simulink model "V2V"  (R2023a)
settings: Solver=FixedStepDiscrete  StartTime=0.0  StopTime=10  FixedStep=0.1  RelTol=1e-3
undefined symbols (not defined in the file): samp_time
(part 1 of 2)
settings Model: Creator=maurizio  LastModifiedBy=alessio
settings SolverCC: MinimalZcImpactIntegration=on
settings DebuggingCC: ReadBeforeWriteMsg=DisableAll  WriteAfterWriteMsg=DisableAll  WriteAfterReadMsg=DisableAll  MultiTaskDSMMsg=none  ModelReferenceSymbolNameMessage=none
settings HardwareCC: TargetBitPerLong=64  TargetBitPerPointer=64  TargetBitPerSizeT=64  TargetBitPerPtrDiffT=64  TargetLongLongMode=on  TargetIntDivRoundTo=Zero  TargetEndianess=LittleEndian  TargetWordSize=64  TargetHWDeviceType=MATLAB Host  ProdEqTarget=off
settings ModelReferenceCC: UpdateModelReferenceTargets=IfOutOfDate
settings SFSimCC: SFSimEcho=off
settings RTWCC: Description=FMU2CS  SystemTargetFile=fmu2cs.tlc  TemplateMakefile=fmu2cs_default_tmf  RTWVerbose=off  RTWUseSimCustomCode=on  BuildConfiguration=Faster Runs
settings CodeAppCC: MaxIdLength=255
settings FMU2CSTargetCC: TargetFcnLib=ansi_tfl_table_tmw.mat  GenFloatMathFcnCalls=NOT IN USE  TargetLangStandard=C99 (ISO)  CodeReplacementLibrary=None  UtilityFuncGeneration=Auto  MultiwordTypeDef=System defined  MultiwordLength=2048  DynamicStringBufferSize=256  GenerateFullHeader=on  InferredTypesCompatibility=off  GenerateSampleERTMain=off  GenerateTestInterfaces=off  ModelReferenceCompliant=on  ParMdlRefBuildCompliant=on  CompOptLevelCompliant=on  ConcurrentExecutionCompliant=on  IncludeMdlTerminateFcn=on  CombineOutputUpdateFcns=on  CombineSignalStateStructs=off  GroupInternalDataByFunction=off  SuppressErrorStatus=off  IncludeFileDelimiter=Auto  ERTCustomFileBanners=off  SupportAbsoluteTime=on  LogVarNameModifier=rt_  MatFileLogging=off  CodeInterfacePackaging=Nonreusable function  PurelyIntegerCode=off  SupportNonFinite=on  SupportComplex=on  SupportContinuousTime=on  SupportNonInlinedSFcns=on  RemoveDisableFunc=off  RemoveResetFunc=off  SupportVariableSizeSignals=off  ParenthesesLevel=Nominal  CastingMode=Nominal  MATLABClassNameForMDSCustomization=Simulink.SoftwareTarget.GRTCustomization  ModelStepFunctionPrototypeControlCompliant=off  CPPClassGenCompliant=on  AutosarCompliant=off  MDXCompliant=off  GRTInterface=off  GenerateAllocFcn=off  UseToolchainInfoCompliant=on  GenerateSharedConstants=on  CoderGroups=[]  AccessMethods=[]  LookupTableObjectStructAxisOrder=1,2,3,4,...  LUTObjectStructOrderExplicitValues=Size,Breakpoints,Table  LUTObjectStructOrderEvenSpacing=Size,Breakpoints,Table  ArrayLayout=Column-major  UnsupportedSFcnMsg=error  ERTHeaderFileRootName=$R$E  ERTSourceFileRootName=$R$E  ERTDataFileRootName=$R_data  OptimizeReductions=off  UseMalloc=off  ExtMode=off  ExtModeStaticAlloc=off  ExtModeTesting=off  ExtModeAutomaticAllocSize=on  ExtModeMaxTrigDuration=10  ExtModeStaticAllocSize=1000000  ExtModeTransport=0  ExtModeMexFile=ext_comm  ExtModeIntrfLevel=Level1  RTWCAPISignals=off  RTWCAPIParams=off  RTWCAPIStates=off  RTWCAPIRootIO=off  GenerateASAP2=off  MultiInstanceErrorCode=Error  CreateModelAfterGeneratingFMU=on  ExportedContent=project  ProjectName=off  AddIcon=off  SaveSourceCodeToFMU=off  AddNativeSimulinkBehavior=off  DataTypeConversion=off  GenerateLinuxBinaryWithWSL=off  FMUType=CS  FMIVersion=2

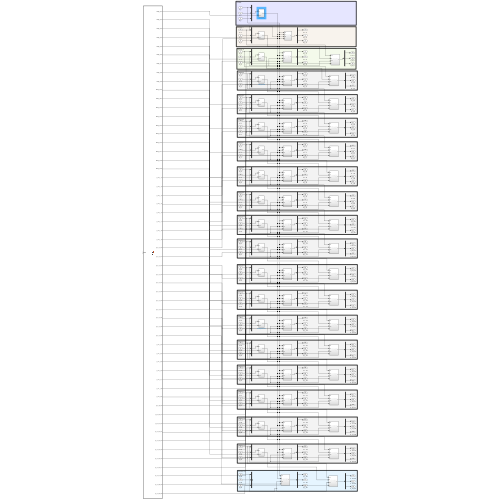
[thumbnail: Simulink's stored preview of the top-level diagram]
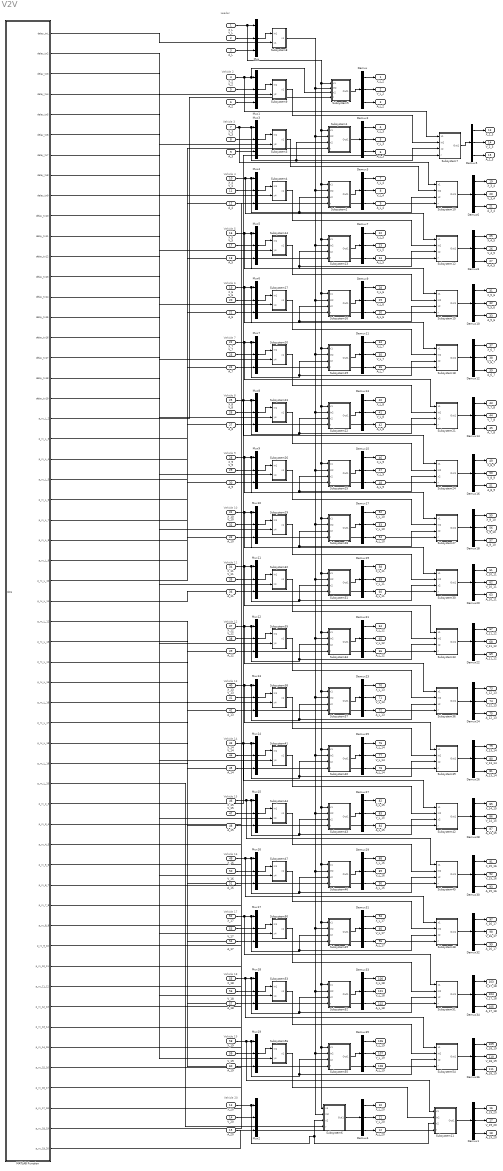
== system V2V ==
  note: Vehicle 3
  note: Vehicle 20
  note: Vehicle 4
  note: Vehicle 2
  note: Leader
  note: Vehicle 5
  note: Vehicle 6
  note: Vehicle 7
  note: Vehicle 8
  note: Vehicle 9
  note: Vehicle 10
  note: Vehicle 11
  note: Vehicle 12
  note: Vehicle 13
  note: Vehicle 14
  note: Vehicle 15
  note: Vehicle 16
  note: Vehicle 17
  note: Vehicle 18
  note: Vehicle 19
  X_L : Inport
  V_L : Inport  Port=2
  A_L : Inport  Port=3
  X_2 : Inport  Port=4
  V_2 : Inport  Port=5
  A_2 : Inport  Port=6
  X_3 : Inport  Port=7
  V_3 : Inport  Port=8
  A_3 : Inport  Port=9
  X_4 : Inport  Port=10
  V_4 : Inport  Port=11
  A_4 : Inport  Port=12
  X_20 : Inport  Port=13
  V_20 : Inport  Port=14
  A_20 : Inport  Port=15
  X_5 : Inport  Port=16
  V_5 : Inport  Port=17
  A_5 : Inport  Port=18
  X_6 : Inport  Port=19
  V_6 : Inport  Port=20
  A_6 : Inport  Port=21
  X_7 : Inport  Port=22
  V_7 : Inport  Port=23
  A_7 : Inport  Port=24
  X_8 : Inport  Port=25
  V_8 : Inport  Port=26
  A_8 : Inport  Port=27
  X_9 : Inport  Port=28
  V_9 : Inport  Port=29
  A_9 : Inport  Port=30
  X_10 : Inport  Port=31
  V_10 : Inport  Port=32
  A_10 : Inport  Port=33
  X_11 : Inport  Port=34
  V_11 : Inport  Port=35
  A_11 : Inport  Port=36
  X_12 : Inport  Port=37
  V_12 : Inport  Port=38
  A_12 : Inport  Port=39
  X_13 : Inport  Port=40
  V_13 : Inport  Port=41
  A_13 : Inport  Port=42
  X_14 : Inport  Port=43
  V_14 : Inport  Port=44
  A_14 : Inport  Port=45
  X_15 : Inport  Port=46
  V_15 : Inport  Port=47
  A_15 : Inport  Port=48
  X_16 : Inport  Port=49
  V_16 : Inport  Port=50
  A_16 : Inport  Port=51
  X_17 : Inport  Port=52
  V_17 : Inport  Port=53
  A_17 : Inport  Port=54
  X_18 : Inport  Port=55
  V_18 : Inport  Port=56
  A_18 : Inport  Port=57
  X_19 : Inport  Port=58
  V_19 : Inport  Port=59
  A_19 : Inport  Port=60
  Demux{,1..36} (37 alike) : Demux  Outputs=3
  MATLAB Function : MATLAB Function  TreatAsAtomicUnit=on  SystemSampleTime=0.1
  Mux{,1..19} (20 alike) : Mux  Inputs=3
  Subsystem1 : Subsystem
  Subsystem10 : Subsystem
  Subsystem11 : Subsystem
  Subsystem12 : Subsystem
  Subsystem13 : Subsystem
  Subsystem14 : Subsystem
  Subsystem15 : Subsystem
  Subsystem16 : Subsystem
  Subsystem17 : Subsystem
  Subsystem18 : Subsystem
  Subsystem19 : Subsystem
  Subsystem2 : Subsystem
  Subsystem20 : Subsystem
  Subsystem21 : Subsystem
  Subsystem22 : Subsystem
  Subsystem23 : Subsystem
  Subsystem24 : Subsystem
  Subsystem25 : Subsystem
  Subsystem26 : Subsystem
  Subsystem27 : Subsystem
  Subsystem28 : Subsystem
  Subsystem29 : Subsystem
  Subsystem3 : Subsystem
  Subsystem30 : Subsystem
  Subsystem31 : Subsystem
  Subsystem32 : Subsystem
  Subsystem33 : Subsystem
  Subsystem34 : Subsystem
  Subsystem35 : Subsystem
  Subsystem36 : Subsystem
  Subsystem37 : Subsystem
  Subsystem38 : Subsystem
  Subsystem39 : Subsystem
  Subsystem4 : Subsystem
  Subsystem40 : Subsystem
  Subsystem41 : Subsystem
  Subsystem42 : Subsystem
  Subsystem43 : Subsystem
  Subsystem44 : Subsystem
  Subsystem45 : Subsystem
  Subsystem46 : Subsystem
  Subsystem47 : Subsystem
  Subsystem48 : Subsystem
  Subsystem49 : Subsystem
  Subsystem5 : Subsystem
  Subsystem50 : Subsystem
  Subsystem51 : Subsystem
  Subsystem52 : Subsystem
  Subsystem53 : Subsystem
  Subsystem54 : Subsystem
  Subsystem55 : Subsystem
  Subsystem56 : Subsystem
  Subsystem6 : Subsystem
  Subsystem7 : Subsystem
  Subsystem8 : Subsystem
  Subsystem9 : Subsystem
  X_L_2 : Outport
  V_L_2 : Outport  Port=2
  A_L_2 : Outport  Port=3
  X_L_3 : Outport  Port=4
  V_L_3 : Outport  Port=5
  A_L_3 : Outport  Port=6
  X_L_4 : Outport  Port=7
  V_L_4 : Outport  Port=8
  A_L_4 : Outport  Port=9
  X_L_20 : Outport  Port=10
  V_L_20 : Outport  Port=11
  A_L_20 : Outport  Port=12
  X_2_3 : Outport  Port=13
  V_2_3 : Outport  Port=14
  A_2_3 : Outport  Port=15
  X_19_20 : Outport  Port=16
  V_19_20 : Outport  Port=17
  A_19_20 : Outport  Port=18
  X_3_4 : Outport  Port=19
  V_3_4 : Outport  Port=20
  A_3_4 : Outport  Port=21
  X_L_5 : Outport  Port=22
  V_L_5 : Outport  Port=23
  A_L_5 : Outport  Port=24
  X_4_5 : Outport  Port=25
  V_4_5 : Outport  Port=26
  A_4_5 : Outport  Port=27
  X_L_6 : Outport  Port=28
  V_L_6 : Outport  Port=29
  A_L_6 : Outport  Port=30
  X_5_6 : Outport  Port=31
  V_5_6 : Outport  Port=32
  A_5_6 : Outport  Port=33
  X_L_7 : Outport  Port=34
  V_L_7 : Outport  Port=35
  A_L_7 : Outport  Port=36
  X_6_7 : Outport  Port=37
  V_6_7 : Outport  Port=38
  A_6_7 : Outport  Port=39
  X_L_8 : Outport  Port=40
  V_L_8 : Outport  Port=41
  A_L_8 : Outport  Port=42
  X_7_8 : Outport  Port=43
  V_7_8 : Outport  Port=44
  A_7_8 : Outport  Port=45
  X_L_9 : Outport  Port=46
  V_L_9 : Outport  Port=47
  A_L_9 : Outport  Port=48
  X_8_9 : Outport  Port=49
  V_8_9 : Outport  Port=50
  A_8_9 : Outport  Port=51
  X_L_10 : Outport  Port=52
  V_L_10 : Outport  Port=53
  A_L_10 : Outport  Port=54
  X_9_10 : Outport  Port=55
  V_9_10 : Outport  Port=56
  A_9_10 : Outport  Port=57
  X_L_11 : Outport  Port=58
  V_L_11 : Outport  Port=59
  A_L_11 : Outport  Port=60
  X_10_11 : Outport  Port=61
  V_10_11 : Outport  Port=62
  A_10_11 : Outport  Port=63
  X_L_12 : Outport  Port=64
  V_L_12 : Outport  Port=65
  A_L_12 : Outport  Port=66
  X_11_12 : Outport  Port=67
  V_11_12 : Outport  Port=68
  A_11_12 : Outport  Port=69
  X_L_13 : Outport  Port=70
  V_L_13 : Outport  Port=71
  A_L_13 : Outport  Port=72
  X_12_13 : Outport  Port=73
  V_12_13 : Outport  Port=74
  A_12_13 : Outport  Port=75
  X_L_14 : Outport  Port=76
  V_L_14 : Outport  Port=77
  A_L_14 : Outport  Port=78
  X_13_14 : Outport  Port=79
  V_13_14 : Outport  Port=80
  A_13_14 : Outport  Port=81
  X_L_15 : Outport  Port=82
  V_L_15 : Outport  Port=83
  A_L_15 : Outport  Port=84
  X_14_15 : Outport  Port=85
  V_14_15 : Outport  Port=86
  A_14_15 : Outport  Port=87
  X_L_16 : Outport  Port=88
  V_L_16 : Outport  Port=89
  A_L_16 : Outport  Port=90
  X_15_16 : Outport  Port=91
  V_15_16 : Outport  Port=92
  A_15_16 : Outport  Port=93
  X_L_17 : Outport  Port=94
  V_L_17 : Outport  Port=95
  A_L_17 : Outport  Port=96
  X_16_17 : Outport  Port=97
  V_16_17 : Outport  Port=98
  A_16_17 : Outport  Port=99
  X_L_18 : Outport  Port=100
  V_L_18 : Outport  Port=101
  A_L_18 : Outport  Port=102
  X_17_18 : Outport  Port=103
  V_17_18 : Outport  Port=104
  A_17_18 : Outport  Port=105
  X_L_19 : Outport  Port=106
  V_L_19 : Outport  Port=107
  A_L_19 : Outport  Port=108
  X_18_19 : Outport  Port=109
  V_18_19 : Outport  Port=110
  A_18_19 : Outport  Port=111
  wires:
  V_L/1 -> Mux/2
  X_L/1 -> Subsystem5/1(x1), Subsystem6/1(x1), Subsystem55/1(x1), Subsystem52/1(x1), Subsystem49/1(x1), Subsystem46/1(x1), Subsystem43/1(x1), Subsystem40/1(x1), Subsystem37/1(x1), Subsystem34/1(x1), Subsystem31/1(x1), Subsystem28/1(x1), Subsystem25/1(x1), Subsystem22/1(x1), Subsystem19/1(x1), Subsystem16/1(x1), Subsystem13/1(x1), Subsystem2/1(x1), Subsystem1/1(x1), Mux/1
  A_L/1 -> Mux/3
  X_2/1 -> Subsystem7/1(x1), Subsystem5/3(x2), Mux1/1
  V_2/1 -> Mux1/2
  A_2/1 -> Mux1/3
  A_3/1 -> Mux3/3
  V_3/1 -> Mux3/2
  X_4/1 -> Subsystem12/1(x1), Subsystem10/3(x2), Subsystem2/3(x2), Mux4/1
  A_4/1 -> Mux4/3
  X_3/1 -> Subsystem10/1(x1), Subsystem7/3(x2), Subsystem1/3(x2), Mux3/1
  V_4/1 -> Mux4/2
  Demux/1 -> X_L_2/1
  Demux/2 -> V_L_2/1
  Demux/3 -> A_L_2/1
  Demux2/1 -> X_L_3/1
  Demux2/3 -> A_L_3/1
  Demux2/2 -> V_L_3/1
  Demux3/3 -> A_L_4/1
  Demux3/1 -> X_L_4/1
  Demux3/2 -> V_L_4/1
  Demux4/2 -> V_L_20/1
  Demux4/1 -> X_L_20/1
  Demux4/3 -> A_L_20/1
  Demux5/3 -> A_2_3/1
  Demux5/2 -> V_2_3/1
  Demux5/1 -> X_2_3/1
  Demux1/3 -> A_19_20/1
  Demux1/2 -> V_19_20/1
  Demux1/1 -> X_19_20/1
  Demux6/3 -> A_3_4/1
  Demux6/2 -> V_3_4/1
  Demux6/1 -> X_3_4/1
  Mux1/1 -> Subsystem9/1(In1)
  Mux3/1 -> Subsystem3/1(In1)
  Mux4/1 -> Subsystem4/1(In1)
  Subsystem5/1(Out1) -> Demux/1
  Mux/1 -> Subsystem8/1(In1)
  Subsystem8/1(x1) -> Subsystem6/2(In2), Subsystem55/2(In2), Subsystem52/2(In2), Subsystem49/2(In2), Subsystem46/2(In2), Subsystem43/2(In2), Subsystem40/2(In2), Subsystem37/2(In2), Subsystem34/2(In2), Subsystem31/2(In2), Subsystem28/2(In2), Subsystem25/2(In2), Subsystem22/2(In2), Subsystem19/2(In2), Subsystem16/2(In2), Subsystem13/2(In2), Subsystem2/2(In2), Subsystem1/2(In2), Subsystem5/2(In2)
  Subsystem2/1(Out1) -> Demux3/1
  Subsystem6/1(Out1) -> Demux4/1
  V_20/1 -> Mux2/2
  A_20/1 -> Mux2/3
  X_20/1 -> Subsystem11/3(x2), Subsystem6/3(x2), Mux2/1
  Subsystem1/1(Out1) -> Demux2/1
  Subsystem7/1(Out1) -> Demux5/1
  Subsystem10/1(Out1) -> Demux6/1
  Subsystem11/1(Out1) -> Demux1/1
  Subsystem9/1(x1) -> Subsystem7/2(In2)
  Subsystem3/1(x1) -> Subsystem10/2(In2)
  MATLAB Function/1(delay_txL) -> Subsystem8/2(y1)
  MATLAB Function/2(delay_tx2) -> Subsystem9/2(y2)
  MATLAB Function/3(delay_tx3) -> Subsystem3/2(y3)
  MATLAB Function/4(delay_tx4) -> Subsystem4/2(y4)
  A_5/1 -> Mux5/3
  Demux7/1 -> X_L_5/1
  Demux7/2 -> V_L_5/1
  Demux7/3 -> A_L_5/1
  Subsystem12/1(Out1) -> Demux8/1
  X_5/1 -> Subsystem15/1(x1), Subsystem12/3(x2), Subsystem13/3(x2), Mux5/1
  Demux8/3 -> A_4_5/1
  V_5/1 -> Mux5/2
  Subsystem13/1(Out1) -> Demux7/1
  Demux8/1 -> X_4_5/1
  Mux5/1 -> Subsystem14/1(In1)
  Demux8/2 -> V_4_5/1
  Subsystem16/1(Out1) -> Demux9/1
  Demux9/3 -> A_L_6/1
  V_6/1 -> Mux6/2
  Demux10/3 -> A_5_6/1
  Demux10/2 -> V_5_6/1
  A_6/1 -> Mux6/3
  X_6/1 -> Subsystem18/1(x1), Subsystem15/3(x2), Subsystem16/3(x2), Mux6/1
  Mux6/1 -> Subsystem17/1(In1)
  Subsystem15/1(Out1) -> Demux10/1
  Demux9/1 -> X_L_6/1
  Demux9/2 -> V_L_6/1
  Demux10/1 -> X_5_6/1
  Subsystem19/1(Out1) -> Demux11/1
  Demux11/3 -> A_L_7/1
  V_7/1 -> Mux7/2
  Demux12/3 -> A_6_7/1
  Demux12/2 -> V_6_7/1
  A_7/1 -> Mux7/3
  X_7/1 -> Subsystem21/1(x1), Subsystem18/3(x2), Subsystem19/3(x2), Mux7/1
  Mux7/1 -> Subsystem20/1(In1)
  Subsystem18/1(Out1) -> Demux12/1
  Demux11/1 -> X_L_7/1
  Demux11/2 -> V_L_7/1
  Demux12/1 -> X_6_7/1
  Subsystem22/1(Out1) -> Demux13/1
  Demux13/3 -> A_L_8/1
  V_8/1 -> Mux8/2
  Demux14/3 -> A_7_8/1
  Demux14/2 -> V_7_8/1
  A_8/1 -> Mux8/3
  X_8/1 -> Subsystem24/1(x1), Subsystem21/3(x2), Subsystem22/3(x2), Mux8/1
  Mux8/1 -> Subsystem23/1(In1)
  Subsystem21/1(Out1) -> Demux14/1
  Demux13/1 -> X_L_8/1
  Demux13/2 -> V_L_8/1
  Demux14/1 -> X_7_8/1
  Subsystem25/1(Out1) -> Demux15/1
  Demux15/3 -> A_L_9/1
  V_9/1 -> Mux9/2
  Demux16/3 -> A_8_9/1
  Demux16/2 -> V_8_9/1
  A_9/1 -> Mux9/3
  X_9/1 -> Subsystem27/1(x1), Subsystem24/3(x2), Subsystem25/3(x2), Mux9/1
  Mux9/1 -> Subsystem26/1(In1)
  Subsystem24/1(Out1) -> Demux16/1
  Demux15/1 -> X_L_9/1
  Demux15/2 -> V_L_9/1
  Demux16/1 -> X_8_9/1
  Subsystem28/1(Out1) -> Demux17/1
  Demux17/3 -> A_L_10/1
  V_10/1 -> Mux10/2
  Demux18/3 -> A_9_10/1
  Demux18/2 -> V_9_10/1
  A_10/1 -> Mux10/3
  X_10/1 -> Subsystem30/1(x1), Subsystem27/3(x2), Subsystem28/3(x2), Mux10/1
  Mux10/1 -> Subsystem29/1(In1)
  Subsystem27/1(Out1) -> Demux18/1
  Demux17/1 -> X_L_10/1
  Demux17/2 -> V_L_10/1
  Demux18/1 -> X_9_10/1
  Subsystem31/1(Out1) -> Demux19/1
  Demux19/3 -> A_L_11/1
  V_11/1 -> Mux11/2
  Demux20/3 -> A_10_11/1
  Demux20/2 -> V_10_11/1
  A_11/1 -> Mux11/3
  X_11/1 -> Subsystem33/1(x1), Subsystem30/3(x2), Subsystem31/3(x2), Mux11/1
  Mux11/1 -> Subsystem32/1(In1)
  Subsystem30/1(Out1) -> Demux20/1
  Demux19/1 -> X_L_11/1
  Demux19/2 -> V_L_11/1
  Demux20/1 -> X_10_11/1
  Subsystem34/1(Out1) -> Demux21/1
  Demux21/3 -> A_L_12/1
  V_12/1 -> Mux12/2
  Demux22/3 -> A_11_12/1
  Demux22/2 -> V_11_12/1
  A_12/1 -> Mux12/3
  X_12/1 -> Subsystem36/1(x1), Subsystem33/3(x2), Subsystem34/3(x2), Mux12/1
  Mux12/1 -> Subsystem35/1(In1)
  Subsystem33/1(Out1) -> Demux22/1
  Demux21/1 -> X_L_12/1
  Demux21/2 -> V_L_12/1
  Demux22/1 -> X_11_12/1
  Subsystem37/1(Out1) -> Demux23/1
  Demux23/3 -> A_L_13/1
  V_13/1 -> Mux13/2
  Demux24/3 -> A_12_13/1
  Demux24/2 -> V_12_13/1
  A_13/1 -> Mux13/3
  X_13/1 -> Subsystem39/1(x1), Subsystem36/3(x2), Subsystem37/3(x2), Mux13/1
  Mux13/1 -> Subsystem38/1(In1)
  Subsystem36/1(Out1) -> Demux24/1
  Demux23/1 -> X_L_13/1
  Demux23/2 -> V_L_13/1
  Demux24/1 -> X_12_13/1
  Subsystem40/1(Out1) -> Demux25/1
  Demux25/3 -> A_L_14/1
  V_14/1 -> Mux14/2
  Demux26/3 -> A_13_14/1
  Demux26/2 -> V_13_14/1
  A_14/1 -> Mux14/3
  X_14/1 -> Subsystem42/1(x1), Subsystem39/3(x2), Subsystem40/3(x2), Mux14/1
  Mux14/1 -> Subsystem41/1(In1)
  Subsystem39/1(Out1) -> Demux26/1
  Demux25/1 -> X_L_14/1
  Demux25/2 -> V_L_14/1
  Demux26/1 -> X_13_14/1
  Subsystem43/1(Out1) -> Demux27/1
  Demux27/3 -> A_L_15/1
  V_15/1 -> Mux15/2
  Demux28/3 -> A_14_15/1
  Demux28/2 -> V_14_15/1
  A_15/1 -> Mux15/3
  X_15/1 -> Subsystem45/1(x1), Subsystem42/3(x2), Subsystem43/3(x2), Mux15/1
  Mux15/1 -> Subsystem44/1(In1)
  Subsystem42/1(Out1) -> Demux28/1
  Demux27/1 -> X_L_15/1
  Demux27/2 -> V_L_15/1
  Demux28/1 -> X_14_15/1
  Subsystem46/1(Out1) -> Demux29/1
  Demux29/3 -> A_L_16/1
  V_16/1 -> Mux16/2
  Demux30/3 -> A_15_16/1
  Demux30/2 -> V_15_16/1
  A_16/1 -> Mux16/3
  X_16/1 -> Subsystem48/1(x1), Subsystem45/3(x2), Subsystem46/3(x2), Mux16/1
  Mux16/1 -> Subsystem47/1(In1)
  Subsystem45/1(Out1) -> Demux30/1
  Demux29/1 -> X_L_16/1
  Demux29/2 -> V_L_16/1
  Demux30/1 -> X_15_16/1
  Subsystem49/1(Out1) -> Demux31/1
  Demux31/3 -> A_L_17/1
  V_17/1 -> Mux17/2
  Demux32/3 -> A_16_17/1
  Demux32/2 -> V_16_17/1
  A_17/1 -> Mux17/3
  X_17/1 -> Subsystem51/1(x1), Subsystem48/3(x2), Subsystem49/3(x2), Mux17/1
  Mux17/1 -> Subsystem50/1(In1)
  Subsystem48/1(Out1) -> Demux32/1
  Demux31/1 -> X_L_17/1
  Demux31/2 -> V_L_17/1
  Demux32/1 -> X_16_17/1
  Subsystem52/1(Out1) -> Demux33/1
  Demux33/3 -> A_L_18/1
  V_18/1 -> Mux18/2
  Demux34/3 -> A_17_18/1
  Demux34/2 -> V_17_18/1
  A_18/1 -> Mux18/3
  X_18/1 -> Subsystem54/1(x1), Subsystem51/3(x2), Subsystem52/3(x2), Mux18/1
  Mux18/1 -> Subsystem53/1(In1)
  Subsystem51/1(Out1) -> Demux34/1
  Demux33/1 -> X_L_18/1
  Demux33/2 -> V_L_18/1
  Demux34/1 -> X_17_18/1
  Subsystem55/1(Out1) -> Demux35/1
  Demux35/3 -> A_L_19/1
  V_19/1 -> Mux19/2
  Demux36/3 -> A_18_19/1
  Demux36/2 -> V_18_19/1
  A_19/1 -> Mux19/3
  X_19/1 -> Subsystem11/1(x1), Subsystem54/3(x2), Subsystem55/3(x2), Mux19/1
  Mux19/1 -> Subsystem56/1(In1)
  Subsystem54/1(Out1) -> Demux36/1
  Demux35/1 -> X_L_19/1
  Demux35/2 -> V_L_19/1
  Demux36/1 -> X_18_19/1
  MATLAB Function/5(delay_tx5) -> Subsystem14/2(y4)
  MATLAB Function/6(delay_tx6) -> Subsystem17/2(y4)
  MATLAB Function/7(delay_tx7) -> Subsystem20/2(y4)
  MATLAB Function/8(delay_tx8) -> Subsystem23/2(y4)
  MATLAB Function/9(delay_tx9) -> Subsystem26/2(y4)
  MATLAB Function/10(delay_tx10) -> Subsystem29/2(y4)
  MATLAB Function/11(delay_tx11) -> Subsystem32/2(y4)
  MATLAB Function/12(delay_tx12) -> Subsystem35/2(y4)
  MATLAB Function/13(delay_tx13) -> Subsystem38/2(y4)
  MATLAB Function/14(delay_tx14) -> Subsystem41/2(y4)
  MATLAB Function/15(delay_tx15) -> Subsystem44/2(y4)
  MATLAB Function/16(delay_tx16) -> Subsystem47/2(y4)
  MATLAB Function/17(delay_tx17) -> Subsystem50/2(y4)
  MATLAB Function/18(delay_tx18) -> Subsystem53/2(y4)
  MATLAB Function/19(delay_tx19) -> Subsystem56/2(y4)
  Subsystem4/1(x1) -> Subsystem12/2(In2)
  Subsystem14/1(x1) -> Subsystem15/2(In2)
  Subsystem17/1(x1) -> Subsystem18/2(In2)
  Subsystem20/1(x1) -> Subsystem21/2(In2)
  Subsystem23/1(x1) -> Subsystem24/2(In2)
  Subsystem26/1(x1) -> Subsystem27/2(In2)
  Subsystem29/1(x1) -> Subsystem30/2(In2)
  Subsystem32/1(x1) -> Subsystem33/2(In2)
  Subsystem35/1(x1) -> Subsystem36/2(In2)
  Subsystem38/1(x1) -> Subsystem39/2(In2)
  Subsystem41/1(x1) -> Subsystem42/2(In2)
  Subsystem44/1(x1) -> Subsystem45/2(In2)
  Subsystem47/1(x1) -> Subsystem48/2(In2)
  Subsystem50/1(x1) -> Subsystem51/2(In2)
  Subsystem53/1(x1) -> Subsystem54/2(In2)
  Subsystem56/1(x1) -> Subsystem11/2(In2)
  MATLAB Function/20(p_rx_L_2) -> Subsystem5/4(r)
  MATLAB Function/21(p_rx_L_3) -> Subsystem1/4(r)
  MATLAB Function/22(p_rx_L_4) -> Subsystem2/4(r)
  MATLAB Function/23(p_rx_L_5) -> Subsystem13/4(r)
  MATLAB Function/24(p_rx_L_6) -> Subsystem16/4(r)
  MATLAB Function/25(p_rx_L_7) -> Subsystem19/4(r)
  MATLAB Function/26(p_rx_L_8) -> Subsystem22/4(r)
  MATLAB Function/27(p_rx_L_9) -> Subsystem25/4(r)
  MATLAB Function/28(p_rx_L_10) -> Subsystem28/4(r)
  MATLAB Function/29(p_rx_L_11) -> Subsystem31/4(r)
  MATLAB Function/30(p_rx_L_12) -> Subsystem34/4(r)
  MATLAB Function/31(p_rx_L_13) -> Subsystem37/4(r)
  MATLAB Function/32(p_rx_L_14) -> Subsystem40/4(r)
  MATLAB Function/33(p_rx_L_15) -> Subsystem43/4(r)
  MATLAB Function/34(p_rx_L_16) -> Subsystem46/4(r)
  MATLAB Function/35(p_rx_L_17) -> Subsystem49/4(r)
  MATLAB Function/36(p_rx_L_18) -> Subsystem52/4(r)
  MATLAB Function/37(p_rx_L_19) -> Subsystem55/4(r)
  MATLAB Function/38(p_rx_L_20) -> Subsystem6/4(r)
  MATLAB Function/56(p_rx_19_20) -> Subsystem11/4(r)
  MATLAB Function/55(p_rx_18_19) -> Subsystem54/4(r)
  MATLAB Function/54(p_rx_17_18) -> Subsystem51/4(r)
  MATLAB Function/53(p_rx_16_17) -> Subsystem48/4(r)
  MATLAB Function/52(p_rx_15_16) -> Subsystem45/4(r)
  MATLAB Function/51(p_rx_14_15) -> Subsystem42/4(r)
  MATLAB Function/50(p_rx_13_14) -> Subsystem39/4(r)
  MATLAB Function/49(p_rx_12_13) -> Subsystem36/4(r)
  MATLAB Function/48(p_rx_11_12) -> Subsystem33/4(r)
  MATLAB Function/39(p_rx_2_3) -> Subsystem7/4(r)
  MATLAB Function/40(p_rx_3_4) -> Subsystem10/4(r)
  MATLAB Function/41(p_rx_4_5) -> Subsystem12/4(r)
  MATLAB Function/42(p_rx_5_6) -> Subsystem15/4(r)
  MATLAB Function/44(p_rx_7_8) -> Subsystem21/4(r)
  MATLAB Function/43(p_rx_6_7) -> Subsystem18/4(r)
  MATLAB Function/45(p_rx_8_9) -> Subsystem24/4(r)
  MATLAB Function/46(p_rx_9_10) -> Subsystem27/4(r)
  MATLAB Function/47(p_rx_10_11) -> Subsystem30/4(r)

== system V2V/Subsystem1 ==
  x1 : Inport
  In2 : Inport  Port=2
  x2 : Inport  Port=3
  r : Inport  Port=4
  Memory : Memory
  Subsystem : Subsystem
  Out1 : Outport
  wires:
  Memory/1 -> Subsystem/3(In3)
  x2/1 -> Subsystem/4(x2)
  Subsystem/1(Out1) -> Out1/1, Memory/1
  x1/1 -> Subsystem/1(x1)
  In2/1 -> Subsystem/2(In2)
  r/1 -> Subsystem/5(r)

== system V2V/Subsystem10 ==
  x1 : Inport
  In2 : Inport  Port=2
  x2 : Inport  Port=3
  r : Inport  Port=4
  Memory : Memory
  Subsystem : Subsystem
  Out1 : Outport
  wires:
  Memory/1 -> Subsystem/3(In3)
  x2/1 -> Subsystem/4(x2)
  Subsystem/1(Out1) -> Out1/1, Memory/1
  x1/1 -> Subsystem/1(x1)
  In2/1 -> Subsystem/2(In2)
  r/1 -> Subsystem/5(r)

== system V2V/Subsystem11 ==
  x1 : Inport
  In2 : Inport  Port=2
  x2 : Inport  Port=3
  r : Inport  Port=4
  Memory : Memory
  Subsystem : Subsystem
  Out1 : Outport
  wires:
  Memory/1 -> Subsystem/3(In3)
  x2/1 -> Subsystem/4(x2)
  Subsystem/1(Out1) -> Out1/1, Memory/1
  x1/1 -> Subsystem/1(x1)
  In2/1 -> Subsystem/2(In2)
  r/1 -> Subsystem/5(r)

== system V2V/Subsystem12 ==
  x1 : Inport
  In2 : Inport  Port=2
  x2 : Inport  Port=3
  r : Inport  Port=4
  Memory : Memory
  Subsystem : Subsystem
  Out1 : Outport
  wires:
  Memory/1 -> Subsystem/3(In3)
  x2/1 -> Subsystem/4(x2)
  Subsystem/1(Out1) -> Out1/1, Memory/1
  x1/1 -> Subsystem/1(x1)
  In2/1 -> Subsystem/2(In2)
  r/1 -> Subsystem/5(r)

== system V2V/Subsystem13 ==
  x1 : Inport
  In2 : Inport  Port=2
  x2 : Inport  Port=3
  r : Inport  Port=4
  Memory : Memory
  Subsystem : Subsystem
  Out1 : Outport
  wires:
  Memory/1 -> Subsystem/3(In3)
  x2/1 -> Subsystem/4(x2)
  Subsystem/1(Out1) -> Out1/1, Memory/1
  x1/1 -> Subsystem/1(x1)
  In2/1 -> Subsystem/2(In2)
  r/1 -> Subsystem/5(r)

== system V2V/Subsystem14 ==
  In1 : Inport
  y4 : Inport  Port=2
  Delay : Delay  DelayLengthSource=Input port  DelayLengthUpperLimit=1000  SampleTime=samp_time
      settings: InputPortMap=u0,p1
  Rate Transition1 : RateTransition  OutPortSampleTimeMultiple=100  OutPortSampleTime=samp_time
  x1 : Outport
  wires:
  y4/1 -> Delay/2
  Rate Transition1/1 -> Delay/1
  Delay/1 -> x1/1
  In1/1 -> Rate Transition1/1

== system V2V/Subsystem15 ==
  x1 : Inport
  In2 : Inport  Port=2
  x2 : Inport  Port=3
  r : Inport  Port=4
  Memory : Memory
  Subsystem : Subsystem
  Out1 : Outport
  wires:
  Memory/1 -> Subsystem/3(In3)
  x2/1 -> Subsystem/4(x2)
  Subsystem/1(Out1) -> Out1/1, Memory/1
  x1/1 -> Subsystem/1(x1)
  In2/1 -> Subsystem/2(In2)
  r/1 -> Subsystem/5(r)

== system V2V/Subsystem16 ==
  x1 : Inport
  In2 : Inport  Port=2
  x2 : Inport  Port=3
  r : Inport  Port=4
  Memory : Memory
  Subsystem : Subsystem
  Out1 : Outport
  wires:
  Memory/1 -> Subsystem/3(In3)
  x2/1 -> Subsystem/4(x2)
  Subsystem/1(Out1) -> Out1/1, Memory/1
  x1/1 -> Subsystem/1(x1)
  In2/1 -> Subsystem/2(In2)
  r/1 -> Subsystem/5(r)

== system V2V/Subsystem17 ==
  In1 : Inport
  y4 : Inport  Port=2
  Delay : Delay  DelayLengthSource=Input port  DelayLengthUpperLimit=1000  SampleTime=samp_time
      settings: InputPortMap=u0,p1
  Rate Transition1 : RateTransition  OutPortSampleTimeMultiple=100  OutPortSampleTime=samp_time
  x1 : Outport
  wires:
  y4/1 -> Delay/2
  Rate Transition1/1 -> Delay/1
  Delay/1 -> x1/1
  In1/1 -> Rate Transition1/1

== system V2V/Subsystem18 ==
  x1 : Inport
  In2 : Inport  Port=2
  x2 : Inport  Port=3
  r : Inport  Port=4
  Memory : Memory
  Subsystem : Subsystem
  Out1 : Outport
  wires:
  Memory/1 -> Subsystem/3(In3)
  x2/1 -> Subsystem/4(x2)
  Subsystem/1(Out1) -> Out1/1, Memory/1
  x1/1 -> Subsystem/1(x1)
  In2/1 -> Subsystem/2(In2)
  r/1 -> Subsystem/5(r)

== system V2V/Subsystem19 ==
  x1 : Inport
  In2 : Inport  Port=2
  x2 : Inport  Port=3
  r : Inport  Port=4
  Memory : Memory
  Subsystem : Subsystem
  Out1 : Outport
  wires:
  Memory/1 -> Subsystem/3(In3)
  x2/1 -> Subsystem/4(x2)
  Subsystem/1(Out1) -> Out1/1, Memory/1
  x1/1 -> Subsystem/1(x1)
  In2/1 -> Subsystem/2(In2)
  r/1 -> Subsystem/5(r)

== system V2V/Subsystem2 ==
  x1 : Inport
  In2 : Inport  Port=2
  x2 : Inport  Port=3
  r : Inport  Port=4
  Memory : Memory
  Subsystem : Subsystem
  Out1 : Outport
  wires:
  Memory/1 -> Subsystem/3(In3)
  x2/1 -> Subsystem/4(x2)
  Subsystem/1(Out1) -> Out1/1, Memory/1
  x1/1 -> Subsystem/1(x1)
  In2/1 -> Subsystem/2(In2)
  r/1 -> Subsystem/5(r)

== system V2V/Subsystem20 ==
  In1 : Inport
  y4 : Inport  Port=2
  Delay : Delay  DelayLengthSource=Input port  DelayLengthUpperLimit=1000  SampleTime=samp_time
      settings: InputPortMap=u0,p1
  Rate Transition1 : RateTransition  OutPortSampleTimeMultiple=100  OutPortSampleTime=samp_time
  x1 : Outport
  wires:
  y4/1 -> Delay/2
  Rate Transition1/1 -> Delay/1
  Delay/1 -> x1/1
  In1/1 -> Rate Transition1/1

== system V2V/Subsystem21 ==
  x1 : Inport
  In2 : Inport  Port=2
  x2 : Inport  Port=3
  r : Inport  Port=4
  Memory : Memory
  Subsystem : Subsystem
  Out1 : Outport
  wires:
  Memory/1 -> Subsystem/3(In3)
  x2/1 -> Subsystem/4(x2)
  Subsystem/1(Out1) -> Out1/1, Memory/1
  x1/1 -> Subsystem/1(x1)
  In2/1 -> Subsystem/2(In2)
  r/1 -> Subsystem/5(r)

== system V2V/Subsystem22 ==
  x1 : Inport
  In2 : Inport  Port=2
  x2 : Inport  Port=3
  r : Inport  Port=4
  Memory : Memory
  Subsystem : Subsystem
  Out1 : Outport
  wires:
  Memory/1 -> Subsystem/3(In3)
  x2/1 -> Subsystem/4(x2)
  Subsystem/1(Out1) -> Out1/1, Memory/1
  x1/1 -> Subsystem/1(x1)
  In2/1 -> Subsystem/2(In2)
  r/1 -> Subsystem/5(r)

== system V2V/Subsystem23 ==
  In1 : Inport
  y4 : Inport  Port=2
  Delay : Delay  DelayLengthSource=Input port  DelayLengthUpperLimit=1000  SampleTime=samp_time
      settings: InputPortMap=u0,p1
  Rate Transition1 : RateTransition  OutPortSampleTimeMultiple=100  OutPortSampleTime=samp_time
  x1 : Outport
  wires:
  y4/1 -> Delay/2
  Rate Transition1/1 -> Delay/1
  Delay/1 -> x1/1
  In1/1 -> Rate Transition1/1

== system V2V/Subsystem24 ==
  x1 : Inport
  In2 : Inport  Port=2
  x2 : Inport  Port=3
  r : Inport  Port=4
  Memory : Memory
  Subsystem : Subsystem
  Out1 : Outport
  wires:
  Memory/1 -> Subsystem/3(In3)
  x2/1 -> Subsystem/4(x2)
  Subsystem/1(Out1) -> Out1/1, Memory/1
  x1/1 -> Subsystem/1(x1)
  In2/1 -> Subsystem/2(In2)
  r/1 -> Subsystem/5(r)

== system V2V/Subsystem25 ==
  x1 : Inport
  In2 : Inport  Port=2
  x2 : Inport  Port=3
  r : Inport  Port=4
  Memory : Memory
  Subsystem : Subsystem
  Out1 : Outport
  wires:
  Memory/1 -> Subsystem/3(In3)
  x2/1 -> Subsystem/4(x2)
  Subsystem/1(Out1) -> Out1/1, Memory/1
  x1/1 -> Subsystem/1(x1)
  In2/1 -> Subsystem/2(In2)
  r/1 -> Subsystem/5(r)

== system V2V/Subsystem26 ==
  In1 : Inport
  y4 : Inport  Port=2
  Delay : Delay  DelayLengthSource=Input port  DelayLengthUpperLimit=1000  SampleTime=samp_time
      settings: InputPortMap=u0,p1
  Rate Transition1 : RateTransition  OutPortSampleTimeMultiple=100  OutPortSampleTime=samp_time
  x1 : Outport
  wires:
  y4/1 -> Delay/2
  Rate Transition1/1 -> Delay/1
  Delay/1 -> x1/1
  In1/1 -> Rate Transition1/1

== system V2V/Subsystem27 ==
  x1 : Inport
  In2 : Inport  Port=2
  x2 : Inport  Port=3
  r : Inport  Port=4
  Memory : Memory
  Subsystem : Subsystem
  Out1 : Outport
  wires:
  Memory/1 -> Subsystem/3(In3)
  x2/1 -> Subsystem/4(x2)
  Subsystem/1(Out1) -> Out1/1, Memory/1
  x1/1 -> Subsystem/1(x1)
  In2/1 -> Subsystem/2(In2)
  r/1 -> Subsystem/5(r)

== system V2V/Subsystem28 ==
  x1 : Inport
  In2 : Inport  Port=2
  x2 : Inport  Port=3
  r : Inport  Port=4
  Memory : Memory
  Subsystem : Subsystem
  Out1 : Outport
  wires:
  Memory/1 -> Subsystem/3(In3)
  x2/1 -> Subsystem/4(x2)
  Subsystem/1(Out1) -> Out1/1, Memory/1
  x1/1 -> Subsystem/1(x1)
  In2/1 -> Subsystem/2(In2)
  r/1 -> Subsystem/5(r)

== system V2V/Subsystem29 ==
  In1 : Inport
  y4 : Inport  Port=2
  Delay : Delay  DelayLengthSource=Input port  DelayLengthUpperLimit=1000  SampleTime=samp_time
      settings: InputPortMap=u0,p1
  Rate Transition1 : RateTransition  OutPortSampleTimeMultiple=100  OutPortSampleTime=samp_time
  x1 : Outport
  wires:
  y4/1 -> Delay/2
  Rate Transition1/1 -> Delay/1
  Delay/1 -> x1/1
  In1/1 -> Rate Transition1/1

== system V2V/Subsystem3 ==
  In1 : Inport
  y3 : Inport  Port=2
  Delay : Delay  DelayLengthSource=Input port  DelayLengthUpperLimit=1000  SampleTime=samp_time
      settings: InputPortMap=u0,p1
  Rate Transition1 : RateTransition  OutPortSampleTimeMultiple=100  OutPortSampleTime=samp_time
  x1 : Outport
  wires:
  y3/1 -> Delay/2
  Rate Transition1/1 -> Delay/1
  Delay/1 -> x1/1
  In1/1 -> Rate Transition1/1

== system V2V/Subsystem30 ==
  x1 : Inport
  In2 : Inport  Port=2
  x2 : Inport  Port=3
  r : Inport  Port=4
  Memory : Memory
  Subsystem : Subsystem
  Out1 : Outport
  wires:
  Memory/1 -> Subsystem/3(In3)
  x2/1 -> Subsystem/4(x2)
  Subsystem/1(Out1) -> Out1/1, Memory/1
  x1/1 -> Subsystem/1(x1)
  In2/1 -> Subsystem/2(In2)
  r/1 -> Subsystem/5(r)

== system V2V/Subsystem31 ==
  x1 : Inport
  In2 : Inport  Port=2
  x2 : Inport  Port=3
  r : Inport  Port=4
  Memory : Memory
  Subsystem : Subsystem
  Out1 : Outport
  wires:
  Memory/1 -> Subsystem/3(In3)
  x2/1 -> Subsystem/4(x2)
  Subsystem/1(Out1) -> Out1/1, Memory/1
  x1/1 -> Subsystem/1(x1)
  In2/1 -> Subsystem/2(In2)
  r/1 -> Subsystem/5(r)

== system V2V/Subsystem32 ==
  In1 : Inport
  y4 : Inport  Port=2
  Delay : Delay  DelayLengthSource=Input port  DelayLengthUpperLimit=1000  SampleTime=samp_time
      settings: InputPortMap=u0,p1
  Rate Transition1 : RateTransition  OutPortSampleTimeMultiple=100  OutPortSampleTime=samp_time
  x1 : Outport
  wires:
  y4/1 -> Delay/2
  Rate Transition1/1 -> Delay/1
  Delay/1 -> x1/1
  In1/1 -> Rate Transition1/1

== system V2V/Subsystem33 ==
  x1 : Inport
  In2 : Inport  Port=2
  x2 : Inport  Port=3
  r : Inport  Port=4
  Memory : Memory
  Subsystem : Subsystem
  Out1 : Outport
  wires:
  Memory/1 -> Subsystem/3(In3)
  x2/1 -> Subsystem/4(x2)
  Subsystem/1(Out1) -> Out1/1, Memory/1
  x1/1 -> Subsystem/1(x1)
  In2/1 -> Subsystem/2(In2)
  r/1 -> Subsystem/5(r)

== system V2V/Subsystem34 ==
  x1 : Inport
  In2 : Inport  Port=2
  x2 : Inport  Port=3
  r : Inport  Port=4
  Memory : Memory
  Subsystem : Subsystem
  Out1 : Outport
  wires:
  Memory/1 -> Subsystem/3(In3)
  x2/1 -> Subsystem/4(x2)
  Subsystem/1(Out1) -> Out1/1, Memory/1
  x1/1 -> Subsystem/1(x1)
  In2/1 -> Subsystem/2(In2)
  r/1 -> Subsystem/5(r)

== system V2V/Subsystem35 ==
  In1 : Inport
  y4 : Inport  Port=2
  Delay : Delay  DelayLengthSource=Input port  DelayLengthUpperLimit=1000  SampleTime=samp_time
      settings: InputPortMap=u0,p1
  Rate Transition1 : RateTransition  OutPortSampleTimeMultiple=100  OutPortSampleTime=samp_time
  x1 : Outport
  wires:
  y4/1 -> Delay/2
  Rate Transition1/1 -> Delay/1
  Delay/1 -> x1/1
  In1/1 -> Rate Transition1/1

== system V2V/Subsystem36 ==
  x1 : Inport
  In2 : Inport  Port=2
  x2 : Inport  Port=3
  r : Inport  Port=4
  Memory : Memory
  Subsystem : Subsystem
  Out1 : Outport
  wires:
  Memory/1 -> Subsystem/3(In3)
  x2/1 -> Subsystem/4(x2)
  Subsystem/1(Out1) -> Out1/1, Memory/1
  x1/1 -> Subsystem/1(x1)
  In2/1 -> Subsystem/2(In2)
  r/1 -> Subsystem/5(r)

== system V2V/Subsystem37 ==
  x1 : Inport
  In2 : Inport  Port=2
  x2 : Inport  Port=3
  r : Inport  Port=4
  Memory : Memory
  Subsystem : Subsystem
  Out1 : Outport
  wires:
  Memory/1 -> Subsystem/3(In3)
  x2/1 -> Subsystem/4(x2)
  Subsystem/1(Out1) -> Out1/1, Memory/1
  x1/1 -> Subsystem/1(x1)
  In2/1 -> Subsystem/2(In2)
  r/1 -> Subsystem/5(r)

== system V2V/Subsystem38 ==
  In1 : Inport
  y4 : Inport  Port=2
  Delay : Delay  DelayLengthSource=Input port  DelayLengthUpperLimit=1000  SampleTime=samp_time
      settings: InputPortMap=u0,p1
  Rate Transition1 : RateTransition  OutPortSampleTimeMultiple=100  OutPortSampleTime=samp_time
  x1 : Outport
  wires:
  y4/1 -> Delay/2
  Rate Transition1/1 -> Delay/1
  Delay/1 -> x1/1
  In1/1 -> Rate Transition1/1

== system V2V/Subsystem39 ==
  x1 : Inport
  In2 : Inport  Port=2
  x2 : Inport  Port=3
  r : Inport  Port=4
  Memory : Memory
  Subsystem : Subsystem
  Out1 : Outport
  wires:
  Memory/1 -> Subsystem/3(In3)
  x2/1 -> Subsystem/4(x2)
  Subsystem/1(Out1) -> Out1/1, Memory/1
  x1/1 -> Subsystem/1(x1)
  In2/1 -> Subsystem/2(In2)
  r/1 -> Subsystem/5(r)

== system V2V/Subsystem4 ==
  In1 : Inport
  y4 : Inport  Port=2
  Delay : Delay  DelayLengthSource=Input port  DelayLengthUpperLimit=1000  SampleTime=samp_time
      settings: InputPortMap=u0,p1
  Rate Transition1 : RateTransition  OutPortSampleTimeMultiple=100  OutPortSampleTime=samp_time
  x1 : Outport
  wires:
  y4/1 -> Delay/2
  Rate Transition1/1 -> Delay/1
  Delay/1 -> x1/1
  In1/1 -> Rate Transition1/1

== system V2V/Subsystem40 ==
  x1 : Inport
  In2 : Inport  Port=2
  x2 : Inport  Port=3
  r : Inport  Port=4
  Memory : Memory
  Subsystem : Subsystem
  Out1 : Outport
  wires:
  Memory/1 -> Subsystem/3(In3)
  x2/1 -> Subsystem/4(x2)
  Subsystem/1(Out1) -> Out1/1, Memory/1
  x1/1 -> Subsystem/1(x1)
  In2/1 -> Subsystem/2(In2)
  r/1 -> Subsystem/5(r)

== system V2V/Subsystem41 ==
  In1 : Inport
  y4 : Inport  Port=2
  Delay : Delay  DelayLengthSource=Input port  DelayLengthUpperLimit=1000  SampleTime=samp_time
      settings: InputPortMap=u0,p1
  Rate Transition1 : RateTransition  OutPortSampleTimeMultiple=100  OutPortSampleTime=samp_time
  x1 : Outport
  wires:
  y4/1 -> Delay/2
  Rate Transition1/1 -> Delay/1
  Delay/1 -> x1/1
  In1/1 -> Rate Transition1/1

== system V2V/Subsystem42 ==
  x1 : Inport
  In2 : Inport  Port=2
  x2 : Inport  Port=3
  r : Inport  Port=4
  Memory : Memory
  Subsystem : Subsystem
  Out1 : Outport
  wires:
  Memory/1 -> Subsystem/3(In3)
  x2/1 -> Subsystem/4(x2)
  Subsystem/1(Out1) -> Out1/1, Memory/1
  x1/1 -> Subsystem/1(x1)
  In2/1 -> Subsystem/2(In2)
  r/1 -> Subsystem/5(r)

== system V2V/Subsystem43 ==
  x1 : Inport
  In2 : Inport  Port=2
  x2 : Inport  Port=3
  r : Inport  Port=4
  Memory : Memory
  Subsystem : Subsystem
  Out1 : Outport
  wires:
  Memory/1 -> Subsystem/3(In3)
  x2/1 -> Subsystem/4(x2)
  Subsystem/1(Out1) -> Out1/1, Memory/1
  x1/1 -> Subsystem/1(x1)
  In2/1 -> Subsystem/2(In2)
  r/1 -> Subsystem/5(r)

== system V2V/Subsystem44 ==
  In1 : Inport
  y4 : Inport  Port=2
  Delay : Delay  DelayLengthSource=Input port  DelayLengthUpperLimit=1000  SampleTime=samp_time
      settings: InputPortMap=u0,p1
  Rate Transition1 : RateTransition  OutPortSampleTimeMultiple=100  OutPortSampleTime=samp_time
  x1 : Outport
  wires:
  y4/1 -> Delay/2
  Rate Transition1/1 -> Delay/1
  Delay/1 -> x1/1
  In1/1 -> Rate Transition1/1

== system V2V/Subsystem45 ==
  x1 : Inport
  In2 : Inport  Port=2
  x2 : Inport  Port=3
  r : Inport  Port=4
  Memory : Memory
  Subsystem : Subsystem
  Out1 : Outport
  wires:
  Memory/1 -> Subsystem/3(In3)
  x2/1 -> Subsystem/4(x2)
  Subsystem/1(Out1) -> Out1/1, Memory/1
  x1/1 -> Subsystem/1(x1)
  In2/1 -> Subsystem/2(In2)
  r/1 -> Subsystem/5(r)

== system V2V/Subsystem46 ==
  x1 : Inport
  In2 : Inport  Port=2
  x2 : Inport  Port=3
  r : Inport  Port=4
  Memory : Memory
  Subsystem : Subsystem
  Out1 : Outport
  wires:
  Memory/1 -> Subsystem/3(In3)
  x2/1 -> Subsystem/4(x2)
  Subsystem/1(Out1) -> Out1/1, Memory/1
  x1/1 -> Subsystem/1(x1)
  In2/1 -> Subsystem/2(In2)
  r/1 -> Subsystem/5(r)

== system V2V/Subsystem47 ==
  In1 : Inport
  y4 : Inport  Port=2
  Delay : Delay  DelayLengthSource=Input port  DelayLengthUpperLimit=1000  SampleTime=samp_time
      settings: InputPortMap=u0,p1
  Rate Transition1 : RateTransition  OutPortSampleTimeMultiple=100  OutPortSampleTime=samp_time
  x1 : Outport
  wires:
  y4/1 -> Delay/2
  Rate Transition1/1 -> Delay/1
  Delay/1 -> x1/1
  In1/1 -> Rate Transition1/1

== system V2V/Subsystem48 ==
  x1 : Inport
  In2 : Inport  Port=2
  x2 : Inport  Port=3
  r : Inport  Port=4
  Memory : Memory
  Subsystem : Subsystem
  Out1 : Outport
  wires:
  Memory/1 -> Subsystem/3(In3)
  x2/1 -> Subsystem/4(x2)
  Subsystem/1(Out1) -> Out1/1, Memory/1
  x1/1 -> Subsystem/1(x1)
  In2/1 -> Subsystem/2(In2)
  r/1 -> Subsystem/5(r)

== system V2V/Subsystem49 ==
  x1 : Inport
  In2 : Inport  Port=2
  x2 : Inport  Port=3
  r : Inport  Port=4
  Memory : Memory
  Subsystem : Subsystem
  Out1 : Outport
  wires:
  Memory/1 -> Subsystem/3(In3)
  x2/1 -> Subsystem/4(x2)
  Subsystem/1(Out1) -> Out1/1, Memory/1
  x1/1 -> Subsystem/1(x1)
  In2/1 -> Subsystem/2(In2)
  r/1 -> Subsystem/5(r)

== system V2V/Subsystem5 ==
  x1 : Inport
  In2 : Inport  Port=2
  x2 : Inport  Port=3
  r : Inport  Port=4
  Memory : Memory
  Subsystem : Subsystem
  Out1 : Outport
  wires:
  Memory/1 -> Subsystem/3(In3)
  x2/1 -> Subsystem/4(x2)
  Subsystem/1(Out1) -> Out1/1, Memory/1
  x1/1 -> Subsystem/1(x1)
  In2/1 -> Subsystem/2(In2)
  r/1 -> Subsystem/5(r)

== system V2V/Subsystem50 ==
  In1 : Inport
  y4 : Inport  Port=2
  Delay : Delay  DelayLengthSource=Input port  DelayLengthUpperLimit=1000  SampleTime=samp_time
      settings: InputPortMap=u0,p1
  Rate Transition1 : RateTransition  OutPortSampleTimeMultiple=100  OutPortSampleTime=samp_time
  x1 : Outport
  wires:
  y4/1 -> Delay/2
  Rate Transition1/1 -> Delay/1
  Delay/1 -> x1/1
  In1/1 -> Rate Transition1/1

== system V2V/Subsystem51 ==
  x1 : Inport
  In2 : Inport  Port=2
  x2 : Inport  Port=3
  r : Inport  Port=4
  Memory : Memory
  Subsystem : Subsystem
  Out1 : Outport
  wires:
  Memory/1 -> Subsystem/3(In3)
  x2/1 -> Subsystem/4(x2)
  Subsystem/1(Out1) -> Out1/1, Memory/1
  x1/1 -> Subsystem/1(x1)
  In2/1 -> Subsystem/2(In2)
  r/1 -> Subsystem/5(r)

== system V2V/Subsystem52 ==
  x1 : Inport
  In2 : Inport  Port=2
  x2 : Inport  Port=3
  r : Inport  Port=4
  Memory : Memory
  Subsystem : Subsystem
  Out1 : Outport
  wires:
  Memory/1 -> Subsystem/3(In3)
  x2/1 -> Subsystem/4(x2)
  Subsystem/1(Out1) -> Out1/1, Memory/1
  x1/1 -> Subsystem/1(x1)
  In2/1 -> Subsystem/2(In2)
  r/1 -> Subsystem/5(r)

== system V2V/Subsystem53 ==
  In1 : Inport
  y4 : Inport  Port=2
  Delay : Delay  DelayLengthSource=Input port  DelayLengthUpperLimit=1000  SampleTime=samp_time
      settings: InputPortMap=u0,p1
  Rate Transition1 : RateTransition  OutPortSampleTimeMultiple=100  OutPortSampleTime=samp_time
  x1 : Outport
  wires:
  y4/1 -> Delay/2
  Rate Transition1/1 -> Delay/1
  Delay/1 -> x1/1
  In1/1 -> Rate Transition1/1

== system V2V/Subsystem54 ==
  x1 : Inport
  In2 : Inport  Port=2
  x2 : Inport  Port=3
  r : Inport  Port=4
  Memory : Memory
  Subsystem : Subsystem
  Out1 : Outport
  wires:
  Memory/1 -> Subsystem/3(In3)
  x2/1 -> Subsystem/4(x2)
  Subsystem/1(Out1) -> Out1/1, Memory/1
  x1/1 -> Subsystem/1(x1)
  In2/1 -> Subsystem/2(In2)
  r/1 -> Subsystem/5(r)

== system V2V/Subsystem55 ==
  x1 : Inport
  In2 : Inport  Port=2
  x2 : Inport  Port=3
  r : Inport  Port=4
  Memory : Memory
  Subsystem : Subsystem
  Out1 : Outport
  wires:
  Memory/1 -> Subsystem/3(In3)
  x2/1 -> Subsystem/4(x2)
  Subsystem/1(Out1) -> Out1/1, Memory/1
  x1/1 -> Subsystem/1(x1)
  In2/1 -> Subsystem/2(In2)
  r/1 -> Subsystem/5(r)

== system V2V/Subsystem56 ==
  In1 : Inport
  y4 : Inport  Port=2
  Delay : Delay  DelayLengthSource=Input port  DelayLengthUpperLimit=1000  SampleTime=samp_time
      settings: InputPortMap=u0,p1
  Rate Transition1 : RateTransition  OutPortSampleTimeMultiple=100  OutPortSampleTime=samp_time
  x1 : Outport
  wires:
  y4/1 -> Delay/2
  Rate Transition1/1 -> Delay/1
  Delay/1 -> x1/1
  In1/1 -> Rate Transition1/1

== system V2V/Subsystem6 ==
  x1 : Inport
  In2 : Inport  Port=2
  x2 : Inport  Port=3
  r : Inport  Port=4
  Memory : Memory
  Subsystem : Subsystem
  Out1 : Outport
  wires:
  Memory/1 -> Subsystem/3(In3)
  x2/1 -> Subsystem/4(x2)
  Subsystem/1(Out1) -> Out1/1, Memory/1
  x1/1 -> Subsystem/1(x1)
  In2/1 -> Subsystem/2(In2)
  r/1 -> Subsystem/5(r)

== system V2V/Subsystem7 ==
  x1 : Inport
  In2 : Inport  Port=2
  x2 : Inport  Port=3
  r : Inport  Port=4
  Memory : Memory
  Subsystem : Subsystem
  Out1 : Outport
  wires:
  Memory/1 -> Subsystem/3(In3)
  x2/1 -> Subsystem/4(x2)
  Subsystem/1(Out1) -> Out1/1, Memory/1
  x1/1 -> Subsystem/1(x1)
  In2/1 -> Subsystem/2(In2)
  r/1 -> Subsystem/5(r)

== system V2V/Subsystem8 ==
  In1 : Inport
  y1 : Inport  Port=2
  Delay : Delay  DelayLengthSource=Input port  DelayLengthUpperLimit=1000  SampleTime=samp_time
      settings: InputPortMap=u0,p1
  Rate Transition1 : RateTransition  OutPortSampleTimeMultiple=100  OutPortSampleTime=samp_time
  x1 : Outport
  wires:
  y1/1 -> Delay/2
  Rate Transition1/1 -> Delay/1
  Delay/1 -> x1/1
  In1/1 -> Rate Transition1/1

== system V2V/Subsystem9 ==
  In1 : Inport
  y2 : Inport  Port=2
  Delay : Delay  DelayLengthSource=Input port  DelayLengthUpperLimit=1000  SampleTime=samp_time
      settings: InputPortMap=u0,p1
  Rate Transition1 : RateTransition  OutPortSampleTimeMultiple=100  OutPortSampleTime=samp_time
  x1 : Outport
  wires:
  y2/1 -> Delay/2
  Rate Transition1/1 -> Delay/1
  Delay/1 -> x1/1
  In1/1 -> Rate Transition1/1

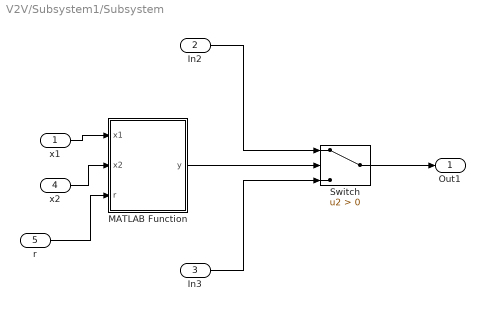
== system V2V/Subsystem1/Subsystem ==
  x1 : Inport
  In2 : Inport  Port=2
  In3 : Inport  Port=3
  x2 : Inport  Port=4
  r : Inport  Port=5
  MATLAB Function : MATLAB Function  TreatAsAtomicUnit=on  SystemSampleTime=0.1
  Switch : Switch  Criteria=u2 > Threshold  SaturateOnIntegerOverflow=off  InputSameDT=off
  Out1 : Outport
  wires:
  x2/1 -> MATLAB Function/2(x2)
  x1/1 -> MATLAB Function/1(x1)
  Switch/1 -> Out1/1
  In2/1 -> Switch/1
  In3/1 -> Switch/3
  MATLAB Function/1(y) -> Switch/2
  r/1 -> MATLAB Function/3(r)

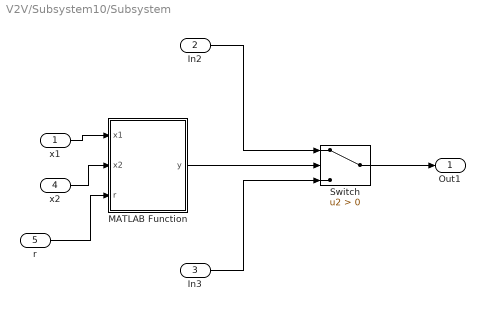
== system V2V/Subsystem10/Subsystem ==
  x1 : Inport
  In2 : Inport  Port=2
  In3 : Inport  Port=3
  x2 : Inport  Port=4
  r : Inport  Port=5
  MATLAB Function : MATLAB Function  TreatAsAtomicUnit=on  SystemSampleTime=0.1
  Switch : Switch  Criteria=u2 > Threshold  SaturateOnIntegerOverflow=off  InputSameDT=off
  Out1 : Outport
  wires:
  x2/1 -> MATLAB Function/2(x2)
  x1/1 -> MATLAB Function/1(x1)
  Switch/1 -> Out1/1
  In2/1 -> Switch/1
  In3/1 -> Switch/3
  MATLAB Function/1(y) -> Switch/2
  r/1 -> MATLAB Function/3(r)

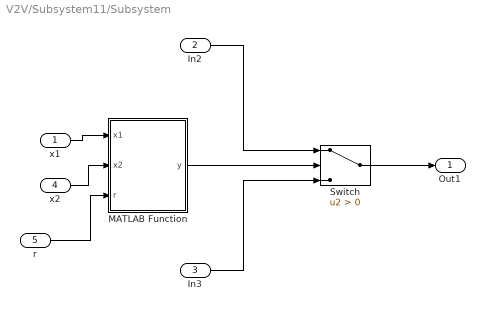
== system V2V/Subsystem11/Subsystem ==
  x1 : Inport
  In2 : Inport  Port=2
  In3 : Inport  Port=3
  x2 : Inport  Port=4
  r : Inport  Port=5
  MATLAB Function : MATLAB Function  TreatAsAtomicUnit=on  SystemSampleTime=0.1
  Switch : Switch  Criteria=u2 > Threshold  SaturateOnIntegerOverflow=off  InputSameDT=off
  Out1 : Outport
  wires:
  x2/1 -> MATLAB Function/2(x2)
  x1/1 -> MATLAB Function/1(x1)
  Switch/1 -> Out1/1
  In2/1 -> Switch/1
  In3/1 -> Switch/3
  MATLAB Function/1(y) -> Switch/2
  r/1 -> MATLAB Function/3(r)

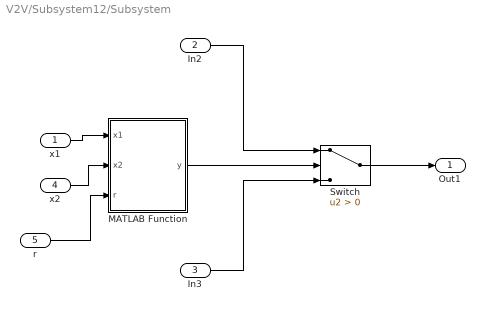
== system V2V/Subsystem12/Subsystem ==
  x1 : Inport
  In2 : Inport  Port=2
  In3 : Inport  Port=3
  x2 : Inport  Port=4
  r : Inport  Port=5
  MATLAB Function : MATLAB Function  TreatAsAtomicUnit=on  SystemSampleTime=0.1
  Switch : Switch  Criteria=u2 > Threshold  SaturateOnIntegerOverflow=off  InputSameDT=off
  Out1 : Outport
  wires:
  x2/1 -> MATLAB Function/2(x2)
  x1/1 -> MATLAB Function/1(x1)
  Switch/1 -> Out1/1
  In2/1 -> Switch/1
  In3/1 -> Switch/3
  MATLAB Function/1(y) -> Switch/2
  r/1 -> MATLAB Function/3(r)

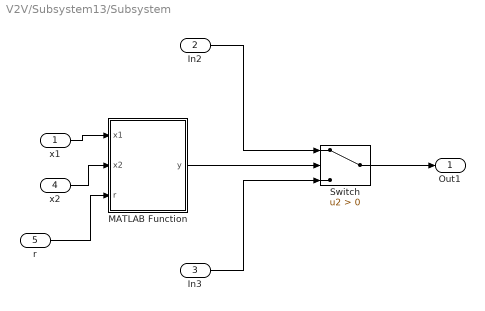
== system V2V/Subsystem13/Subsystem ==
  x1 : Inport
  In2 : Inport  Port=2
  In3 : Inport  Port=3
  x2 : Inport  Port=4
  r : Inport  Port=5
  MATLAB Function : MATLAB Function  TreatAsAtomicUnit=on  SystemSampleTime=0.1
  Switch : Switch  Criteria=u2 > Threshold  SaturateOnIntegerOverflow=off  InputSameDT=off
  Out1 : Outport
  wires:
  x2/1 -> MATLAB Function/2(x2)
  x1/1 -> MATLAB Function/1(x1)
  Switch/1 -> Out1/1
  In2/1 -> Switch/1
  In3/1 -> Switch/3
  MATLAB Function/1(y) -> Switch/2
  r/1 -> MATLAB Function/3(r)

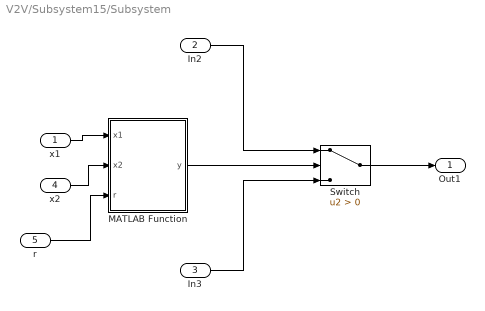
== system V2V/Subsystem15/Subsystem ==
  x1 : Inport
  In2 : Inport  Port=2
  In3 : Inport  Port=3
  x2 : Inport  Port=4
  r : Inport  Port=5
  MATLAB Function : MATLAB Function  TreatAsAtomicUnit=on  SystemSampleTime=0.1
  Switch : Switch  Criteria=u2 > Threshold  SaturateOnIntegerOverflow=off  InputSameDT=off
  Out1 : Outport
  wires:
  x2/1 -> MATLAB Function/2(x2)
  x1/1 -> MATLAB Function/1(x1)
  Switch/1 -> Out1/1
  In2/1 -> Switch/1
  In3/1 -> Switch/3
  MATLAB Function/1(y) -> Switch/2
  r/1 -> MATLAB Function/3(r)

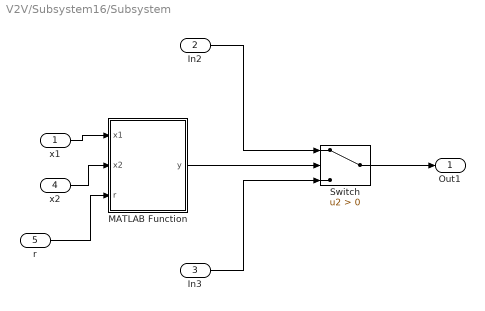
== system V2V/Subsystem16/Subsystem ==
  x1 : Inport
  In2 : Inport  Port=2
  In3 : Inport  Port=3
  x2 : Inport  Port=4
  r : Inport  Port=5
  MATLAB Function : MATLAB Function  TreatAsAtomicUnit=on  SystemSampleTime=0.1
  Switch : Switch  Criteria=u2 > Threshold  SaturateOnIntegerOverflow=off  InputSameDT=off
  Out1 : Outport
  wires:
  x2/1 -> MATLAB Function/2(x2)
  x1/1 -> MATLAB Function/1(x1)
  Switch/1 -> Out1/1
  In2/1 -> Switch/1
  In3/1 -> Switch/3
  MATLAB Function/1(y) -> Switch/2
  r/1 -> MATLAB Function/3(r)

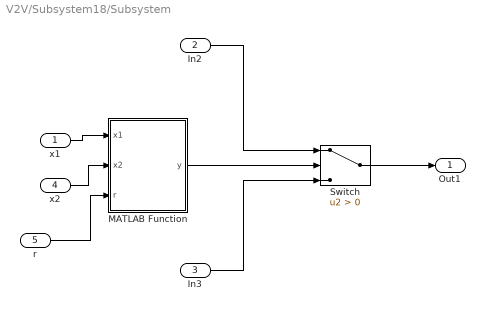
== system V2V/Subsystem18/Subsystem ==
  x1 : Inport
  In2 : Inport  Port=2
  In3 : Inport  Port=3
  x2 : Inport  Port=4
  r : Inport  Port=5
  MATLAB Function : MATLAB Function  TreatAsAtomicUnit=on  SystemSampleTime=0.1
  Switch : Switch  Criteria=u2 > Threshold  SaturateOnIntegerOverflow=off  InputSameDT=off
  Out1 : Outport
  wires:
  x2/1 -> MATLAB Function/2(x2)
  x1/1 -> MATLAB Function/1(x1)
  Switch/1 -> Out1/1
  In2/1 -> Switch/1
  In3/1 -> Switch/3
  MATLAB Function/1(y) -> Switch/2
  r/1 -> MATLAB Function/3(r)

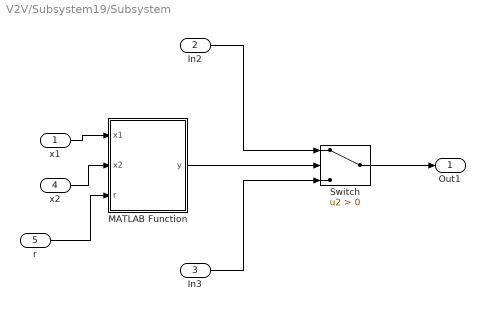
== system V2V/Subsystem19/Subsystem ==
  x1 : Inport
  In2 : Inport  Port=2
  In3 : Inport  Port=3
  x2 : Inport  Port=4
  r : Inport  Port=5
  MATLAB Function : MATLAB Function  TreatAsAtomicUnit=on  SystemSampleTime=0.1
  Switch : Switch  Criteria=u2 > Threshold  SaturateOnIntegerOverflow=off  InputSameDT=off
  Out1 : Outport
  wires:
  x2/1 -> MATLAB Function/2(x2)
  x1/1 -> MATLAB Function/1(x1)
  Switch/1 -> Out1/1
  In2/1 -> Switch/1
  In3/1 -> Switch/3
  MATLAB Function/1(y) -> Switch/2
  r/1 -> MATLAB Function/3(r)

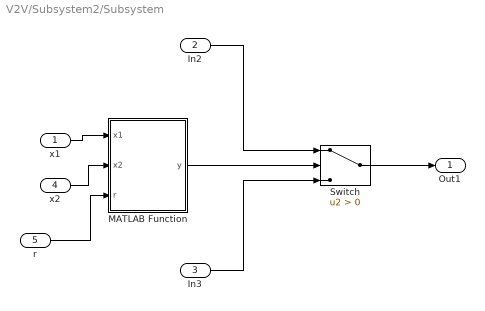
== system V2V/Subsystem2/Subsystem ==
  x1 : Inport
  In2 : Inport  Port=2
  In3 : Inport  Port=3
  x2 : Inport  Port=4
  r : Inport  Port=5
  MATLAB Function : MATLAB Function  TreatAsAtomicUnit=on  SystemSampleTime=0.1
  Switch : Switch  Criteria=u2 > Threshold  SaturateOnIntegerOverflow=off  InputSameDT=off
  Out1 : Outport
  wires:
  x2/1 -> MATLAB Function/2(x2)
  x1/1 -> MATLAB Function/1(x1)
  Switch/1 -> Out1/1
  In2/1 -> Switch/1
  In3/1 -> Switch/3
  MATLAB Function/1(y) -> Switch/2
  r/1 -> MATLAB Function/3(r)

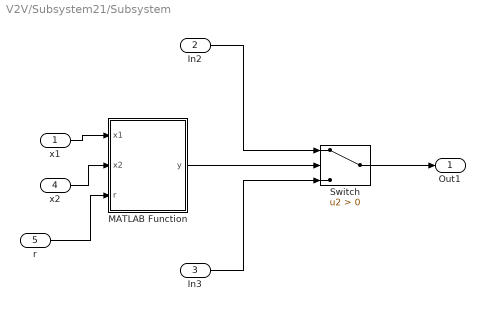
== system V2V/Subsystem21/Subsystem ==
  x1 : Inport
  In2 : Inport  Port=2
  In3 : Inport  Port=3
  x2 : Inport  Port=4
  r : Inport  Port=5
  MATLAB Function : MATLAB Function  TreatAsAtomicUnit=on  SystemSampleTime=0.1
  Switch : Switch  Criteria=u2 > Threshold  SaturateOnIntegerOverflow=off  InputSameDT=off
  Out1 : Outport
  wires:
  x2/1 -> MATLAB Function/2(x2)
  x1/1 -> MATLAB Function/1(x1)
  Switch/1 -> Out1/1
  In2/1 -> Switch/1
  In3/1 -> Switch/3
  MATLAB Function/1(y) -> Switch/2
  r/1 -> MATLAB Function/3(r)

== system V2V/Subsystem22/Subsystem ==
  x1 : Inport
  In2 : Inport  Port=2
  In3 : Inport  Port=3
  x2 : Inport  Port=4
  r : Inport  Port=5
  MATLAB Function : MATLAB Function  TreatAsAtomicUnit=on  SystemSampleTime=0.1
  Switch : Switch  Criteria=u2 > Threshold  SaturateOnIntegerOverflow=off  InputSameDT=off
  Out1 : Outport
  wires:
  x2/1 -> MATLAB Function/2(x2)
  x1/1 -> MATLAB Function/1(x1)
  Switch/1 -> Out1/1
  In2/1 -> Switch/1
  In3/1 -> Switch/3
  MATLAB Function/1(y) -> Switch/2
  r/1 -> MATLAB Function/3(r)

== system V2V/Subsystem24/Subsystem ==
  x1 : Inport
  In2 : Inport  Port=2
  In3 : Inport  Port=3
  x2 : Inport  Port=4
  r : Inport  Port=5
  MATLAB Function : MATLAB Function  TreatAsAtomicUnit=on  SystemSampleTime=0.1
  Switch : Switch  Criteria=u2 > Threshold  SaturateOnIntegerOverflow=off  InputSameDT=off
  Out1 : Outport
  wires:
  x2/1 -> MATLAB Function/2(x2)
  x1/1 -> MATLAB Function/1(x1)
  Switch/1 -> Out1/1
  In2/1 -> Switch/1
  In3/1 -> Switch/3
  MATLAB Function/1(y) -> Switch/2
  r/1 -> MATLAB Function/3(r)

== system V2V/Subsystem25/Subsystem ==
  x1 : Inport
  In2 : Inport  Port=2
  In3 : Inport  Port=3
  x2 : Inport  Port=4
  r : Inport  Port=5
  MATLAB Function : MATLAB Function  TreatAsAtomicUnit=on  SystemSampleTime=0.1
  Switch : Switch  Criteria=u2 > Threshold  SaturateOnIntegerOverflow=off  InputSameDT=off
  Out1 : Outport
  wires:
  x2/1 -> MATLAB Function/2(x2)
  x1/1 -> MATLAB Function/1(x1)
  Switch/1 -> Out1/1
  In2/1 -> Switch/1
  In3/1 -> Switch/3
  MATLAB Function/1(y) -> Switch/2
  r/1 -> MATLAB Function/3(r)

== system V2V/Subsystem27/Subsystem ==
  x1 : Inport
  In2 : Inport  Port=2
  In3 : Inport  Port=3
  x2 : Inport  Port=4
  r : Inport  Port=5
  MATLAB Function : MATLAB Function  TreatAsAtomicUnit=on  SystemSampleTime=0.1
  Switch : Switch  Criteria=u2 > Threshold  SaturateOnIntegerOverflow=off  InputSameDT=off
  Out1 : Outport
  wires:
  x2/1 -> MATLAB Function/2(x2)
  x1/1 -> MATLAB Function/1(x1)
  Switch/1 -> Out1/1
  In2/1 -> Switch/1
  In3/1 -> Switch/3
  MATLAB Function/1(y) -> Switch/2
  r/1 -> MATLAB Function/3(r)
